simulink subsystem "subsistema_electrico_corriente_I_0s"  (R2023b)
settings: Solver=VariableStepAuto  StartTime=0.0  StopTime=10.0  RelTol=1e-3
undefined symbols (not defined in the file or in its folder): L_ls
settings Model: Creator=nicol  LastModifiedBy=Julya

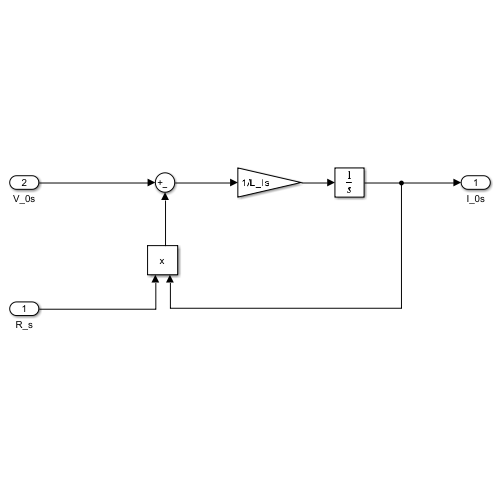
[thumbnail: Simulink's stored preview of the top-level diagram]
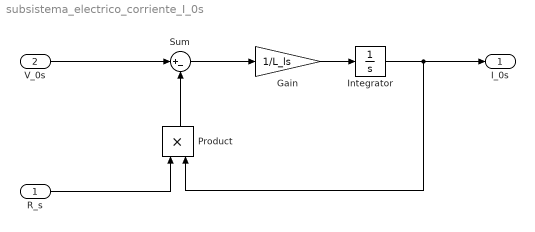
== system subsistema_electrico_corriente_I_0s ==
  R_s : Inport
  V_0s : Inport  Port=2
  Gain : Gain  Gain=1/L_ls
  Integrator : Integrator
  Product : Product
  Sum : Sum  Inputs=|+-
  I_0s : Outport
  wires:
  V_0s/1 -> Sum/1
  Sum/1 -> Gain/1
  Gain/1 -> Integrator/1
  Integrator/1 -> Product/2, I_0s/1
  R_s/1 -> Product/1
  Product/1 -> Sum/2
